simulink model "model"  (R2022a)
settings: Solver=VariableStepAuto  StartTime=0.0  StopTime=10.0  RelTol=1e-3
values from neighbouring files (symbols this model uses):
  dy_0 = 0    [config.m]
  K_1 = -1    [tasks.m]
  K_2 = -1    [tasks.m]
  T = 0.2    [config.m]
  y_0 = 1    [config.m]
settings Model: Creator=Vvlad  LastModifiedBy=Vvlad

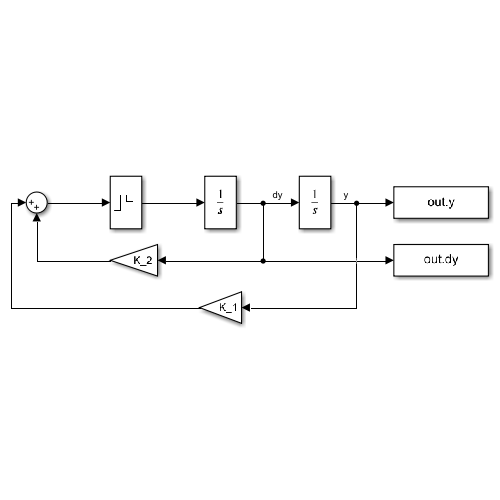
[thumbnail: Simulink's stored preview of the top-level diagram]
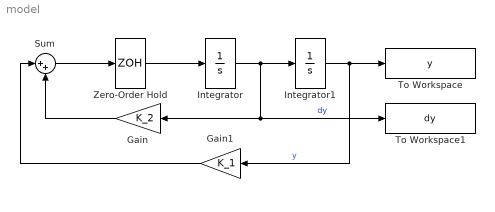
== system model ==
  Gain : Gain  Gain=K_2
  Gain1 : Gain  Gain=K_1
  Integrator : Integrator  InitialCondition=dy_0
  Integrator1 : Integrator  InitialCondition=y_0
  Sum : Sum  Inputs=|++
  To Workspace : ToWorkspace  VariableName=y  SampleTime=-1
  To Workspace1 : ToWorkspace  VariableName=dy  SampleTime=-1
  Zero-Order Hold : ZeroOrderHold  SampleTime=T
  wires:
  Zero-Order Hold/1 -> Integrator/1
  Sum/1 -> Zero-Order Hold/1
  Gain/1 -> Sum/2
  Gain1/1 -> Sum/1
  Integrator/1 -> To Workspace1/1, Gain/1, Integrator1/1  "dy"
  Integrator1/1 -> To Workspace/1, Gain1/1  "y"
